simulink model "Clack_Park"  (R2021b)
settings: Solver=VariableStepAuto  StartTime=0.0  StopTime=1  RelTol=1e-3
libraries: simulink x1
settings Model: Creator=SZQC  LastModifiedBy=SZQC

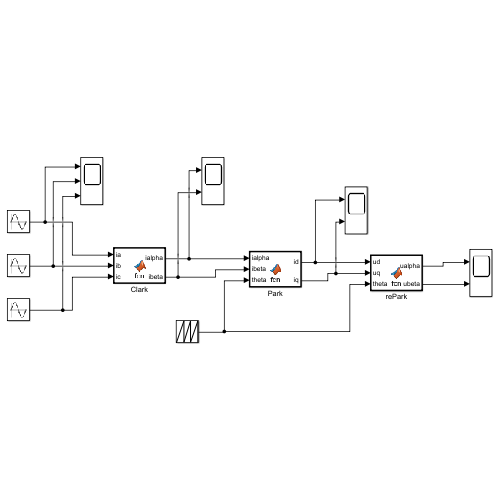
[thumbnail: Simulink's stored preview of the top-level diagram]
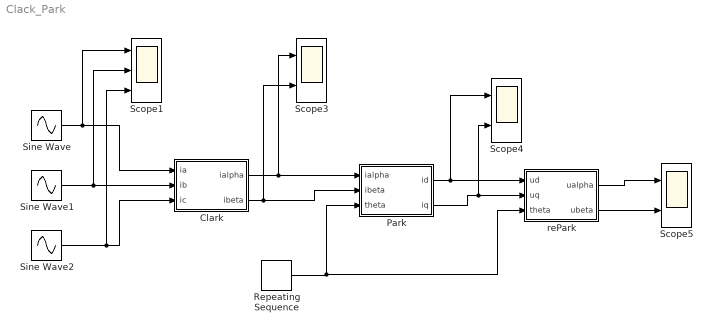
== system Clack_Park ==
  Clark : MATLAB Function  TreatAsAtomicUnit=on
  Park : MATLAB Function  TreatAsAtomicUnit=on
  Repeating Sequence : simulink/Sources/Repeating Sequence  rep_seq_t=[0 0.1]  rep_seq_y=[0 2*pi]
  Scope1 : Scope  NumInputPorts=3
  Scope3 : Scope  NumInputPorts=2
  Scope4 : Scope  NumInputPorts=2
  Scope5 : Scope  NumInputPorts=2
  Sine Wave : Sin  Amplitude=24  Frequency=3.2*pi  SampleTime=0
  Sine Wave1 : Sin  Amplitude=24  Frequency=3.2*pi  Phase=2*pi/3  SampleTime=0
  Sine Wave2 : Sin  Amplitude=24  Frequency=3.2*pi  Phase=2*pi*2/3  SampleTime=0
  rePark : MATLAB Function  TreatAsAtomicUnit=on
  wires:
  Sine Wave/1 -> Scope1/1, Clark/1(ia)
  Sine Wave1/1 -> Scope1/2, Clark/2(ib)
  Sine Wave2/1 -> Scope1/3, Clark/3(ic)
  Clark/1(ialpha) -> Scope3/1, Park/1(ialpha)
  Clark/2(ibeta) -> Scope3/2, Park/2(ibeta)
  Repeating Sequence/1 -> rePark/3(theta), Park/3(theta)
  Park/1(id) -> Scope4/1, rePark/1(ud)
  Park/2(iq) -> Scope4/2, rePark/2(uq)
  rePark/1(ualpha) -> Scope5/1
  rePark/2(ubeta) -> Scope5/2

== matlab function Clack_Park/Park ==
  data: ialpha input; id output; ibeta input; theta input; iq output
function [id,iq] = fcn(ialpha,ibeta,theta)
id=ialpha*cos(theta)+ibeta*sin(theta);
iq=-ialpha*sin(theta)+ibeta*cos(theta);

== matlab function Clack_Park/Clark ==
  data: ia input; ialpha output; ib input; ic input; ibeta output
function [ialpha,ibeta]= fcn(ia,ib,ic)
ialpha=(ia-(ib+ic)/2)*2/3;
ibeta=((ib-ic)*sqrt(3)/2)*2/3;

== matlab function Clack_Park/rePark ==
  data: ud input; ualpha output; uq input; theta input; ubeta output
function [ualpha,ubeta] = fcn(ud,uq,theta)
ualpha=ud*cos(theta)-uq*sin(theta);
ubeta=ud*sin(theta)+uq*cos(theta);
